simulink model "CryoDetXray"  (R2016b)
settings: Solver=ode45  StartTime=0.0  StopTime=10e-5  MaxStep=Tclk/4  RelTol=1e-3
values from neighbouring files (symbols this model uses):
  Fclk = Fadc    (= 307200000)    [setupCryoFPGAxray.m]
  Tclk = 1/Fclk    (= 3.25520833333e-09)    [setupCryoFPGAxray.m]
undefined symbols (not defined in the file or in its folder): AXI4, Lite, lpf, Naxi, xlipgetpartsetting
libraries: xbsIndex_r4 x1091, CryoDetLib x68, simulink x4, hdlsllib x1
(part 6 of 8)

== system CryoDetXray/DspCore/AdcDac 0/dF1 ==
  note: negate Q component to form conjugate
  note: "Now bandwidth is included in eta'
  note: definition of eta' changed so that now delta(F) = real part of eta'*Sig*conj(Ref)
      | SS 27 Spe 2017
  note: diagnostics
  note: latency 1
  note: pick a channel for diagnostics
  note: sig0
  note: conj(Ref0)
  note: Match latencies
  note: dF1
  note: Ref
  note: Sig
  note: Frequency error dF = Re(eta'*Ref'*Sig)
      | where eta' is like a phase and amplitude calibration including the phase determined by the 2 sidebands and amplitude determined by the reference central line and bandwidth
      |
      | get channel ID
      | fetch eta'
      | calc dF
  note: latency 12
  note: latency 12
  In1 : Inport
  Bus Creator : BusCreator  Inputs=2
  Bus Selector : BusSelector  OutputSignals=channel,Sig&Ref
  Bus Selector1 : BusSelector  OutputSignals=SignalQ&I,ReferenceQ&I
  Bus Selector2 : BusSelector  OutputSignals=refQ,refI
  Bus Selector3 : BusSelector  OutputSignals=sigQ,sigI
  Bus Selector4 : BusSelector  OutputSignals=imEta,reEta
  CMult : xbsIndex_r4/CMult  const=-1  gui_display_data_type=Fixed-point  const_n_bits=16  const_bin_pt=15  float_type=Single  exp_bits=8  fraction_bits=24  en=off  latency=1  precision=User Defined  arith_type="Signed  (2's comp)"  n_bits=16  bin_pt=16  quantization=Truncate  overflow=Saturate  use_behavioral_HDL=on  mem_type=Distributed RAM  pipeline=off  dbl_ovrd=off  block_type=cmult
  Chan Synch scope : Scope  Commented=on  NumInputPorts=2
  "Complex Multiplier 6.0 " : xbsIndex_r4/Complex Multiplier 6.0   hasatlast=off  hasatuser=off  atuserwidth=1  hasbtlast=off  hasbtuser=on  btuserwidth=4  multtype=Use_Mults  optimizegoal=Performance  flowcontrol=NonBlocking  outputwidth=20  roundmode=Truncate  hasctrltlast=off  hasctrltuser=off  ctrltuserwidth=1  outtlastbehv=Null  latencyconfig=Manual  minimumlatency=8  aclken=off  aresetn=off  trim_axipin_name=on  simulation_type=hybrid_sim  simulation_model=sysgen:cmpy_v6_0  data_path_portlist={ 's_axis_a_tdata_real', 's_axis_a_tdata_imag', 's_axis_b_tdata_real', 's_axis_b_tdata_imag', 's_axis_ctrl_tdata_rounding_bit', 'm_axis_dout_tdata_real', 'm_axis_dout_tdata_imag' }  aportwidth=63  bportwidth=63  ip_name=Complex Multiplier  ip_version=6.0  dsptool_ready=true  ipcore_usecache=true  ipcore_useipmodelcache=true  ipcore_verbose=false  ipcore_latency_parameter='minimumlatency'  wrapper_available=true  port_translation_map={ 'aclken' => 'en', 'aresetn' => 'rst'}  block_type=cmpy_v6_0
  Complex Multiplier 6.0 1 : xbsIndex_r4/Complex Multiplier 6.0   hasatlast=off  hasatuser=on  atuserwidth=4  hasbtlast=off  hasbtuser=off  btuserwidth=1  multtype=Use_Mults  optimizegoal=Performance  flowcontrol=NonBlocking  outputwidth=34  roundmode=Truncate  hasctrltlast=off  hasctrltuser=off  ctrltuserwidth=1  outtlastbehv=Null  latencyconfig=Manual  minimumlatency=12  aclken=off  aresetn=off  trim_axipin_name=on  simulation_type=hybrid_sim  simulation_model=sysgen:cmpy_v6_0  data_path_portlist={ 's_axis_a_tdata_real', 's_axis_a_tdata_imag', 's_axis_b_tdata_real', 's_axis_b_tdata_imag', 's_axis_ctrl_tdata_rounding_bit', 'm_axis_dout_tdata_real', 'm_axis_dout_tdata_imag' }  aportwidth=63  bportwidth=63  ip_name=Complex Multiplier  ip_version=6.0  dsptool_ready=true  ipcore_usecache=true  ipcore_useipmodelcache=true  ipcore_verbose=false  ipcore_latency_parameter='minimumlatency'  wrapper_available=true  port_translation_map={ 'aclken' => 'en', 'aresetn' => 'rst'}  block_type=cmpy_v6_0
  Constant : xbsIndex_r4/Constant  const=0  gui_display_data_type=Fixed-point  arith_type=Unsigned  n_bits=4  bin_pt=0  preci_type=Single  exp_width=8  frac_width=24  explicit_period=off  period=1  equ=P=C  opselect=C  inp2=PCIN>>17  opr=+  inp1=P  carry=CIN  dbl_ovrd=off  block_type=constant
  Constant1 : xbsIndex_r4/Constant  const=1  gui_display_data_type=Fixed-point  arith_type=Unsigned  n_bits=4  bin_pt=0  preci_type=Single  exp_width=8  frac_width=24  explicit_period=off  period=1  equ=P=C  opselect=C  inp2=PCIN>>17  opr=+  inp1=P  carry=CIN  dbl_ovrd=off  block_type=constant
  Constant2 : xbsIndex_r4/Constant  const=1.0  gui_display_data_type=Boolean  arith_type=Boolean  n_bits=16  bin_pt=14  preci_type=Single  exp_width=8  frac_width=24  explicit_period=on  period=Tclk  equ=P=C  opselect=C  inp2=PCIN>>17  opr=+  inp1=P  carry=CIN  dbl_ovrd=off  block_type=constant
  Constant3 : xbsIndex_r4/Constant  const=0  gui_display_data_type=Fixed-point  arith_type=Unsigned  n_bits=4  bin_pt=0  preci_type=Single  exp_width=8  frac_width=24  explicit_period=off  period=1  equ=P=C  opselect=C  inp2=PCIN>>17  opr=+  inp1=P  carry=CIN  dbl_ovrd=off  block_type=constant
  Constant4 : Constant  Value=0
  Convert : xbsIndex_r4/Convert  gui_display_data_type=Fixed-point  arith_type="Signed  (2's comp)"  n_bits=16  bin_pt=16  float_type=Single  exp_bits=8  fraction_bits=24  quantization=Truncate  overflow=Wrap  en=off  latency=1  pipeline=on  dbl_ovrd=off  block_type=convert
  Convert1 : xbsIndex_r4/Convert  gui_display_data_type=Fixed-point  arith_type="Signed  (2's comp)"  n_bits=16  bin_pt=16  float_type=Single  exp_bits=8  fraction_bits=24  quantization=Truncate  overflow=Wrap  en=off  latency=1  pipeline=on  dbl_ovrd=off  block_type=convert
  Convert3 : xbsIndex_r4/Convert  gui_display_data_type=Fixed-point  arith_type="Signed  (2's comp)"  n_bits=16  bin_pt=16  float_type=Single  exp_bits=8  fraction_bits=24  quantization=Truncate  overflow=Wrap  en=off  latency=1  pipeline=on  dbl_ovrd=off  block_type=convert
  Convert4 : xbsIndex_r4/Convert  gui_display_data_type=Fixed-point  arith_type="Signed  (2's comp)"  n_bits=32  bin_pt=30  float_type=Single  exp_bits=8  fraction_bits=24  quantization="Round  (unbiased: +/- Inf)"  overflow=Saturate  en=off  latency=1  pipeline=off  dbl_ovrd=off  block_type=convert
  Convert6 : xbsIndex_r4/Convert  gui_display_data_type=Fixed-point  arith_type="Signed  (2's comp)"  n_bits=16  bin_pt=14  float_type=Single  exp_bits=8  fraction_bits=24  quantization=Truncate  overflow=Wrap  en=off  latency=1  pipeline=on  dbl_ovrd=off  block_type=convert
  Convert7 : xbsIndex_r4/Convert  gui_display_data_type=Fixed-point  arith_type="Signed  (2's comp)"  n_bits=16  bin_pt=14  float_type=Single  exp_bits=8  fraction_bits=24  quantization=Truncate  overflow=Wrap  en=off  latency=1  pipeline=on  dbl_ovrd=off  block_type=convert
  Delay{1,5..6,10..11} (5 alike) : xbsIndex_r4/Delay  rst=off  infoeditControl=Selection of Reset will increase slice count due to use of real FFs and instead of SRLs  en=off  latency=1  reg_retiming=on  dbl_ovrd=off  block_type=delay
  Delay3 : xbsIndex_r4/Delay  rst=off  infoeditControl=Selection of Reset will increase slice count due to use of real FFs and instead of SRLs  en=off  latency=12  reg_retiming=on  dbl_ovrd=off  block_type=delay
  Delay4 : xbsIndex_r4/Delay  rst=off  infoeditControl=Selection of Reset will increase slice count due to use of real FFs and instead of SRLs  en=off  latency=6  reg_retiming=on  dbl_ovrd=off  block_type=delay
  Freq Error : Scope
  Gain3 : Gain  Gain=Fclk/1e6
  Gain4 : Gain  Gain=Fclk/1e6
  Gateway Out{1..7,9} (8 alike) : xbsIndex_r4/Gateway Out  inherit_from_input=off  hdl_port=off  rows=1  columns=1  UseAsDAC=off  DACChannel='1'  interface=None  automatic_assignment=on  address_offset=hex2dec('00')  intf_name=''  intf_description=''  timing_constraint=None  locs_specified=off  LOCs={}  io_standard={}  block_type=gatewayout
  Im SigXRef 0 : Display
  Re SigXRef 0 : Display
  Register{,1..3} (4 alike) : xbsIndex_r4/Register  init=0  rst=off  en=on  dbl_ovrd=off  block_type=register
  Register{4..7} (4 alike) : xbsIndex_r4/Register  init=0  rst=off  en=off  dbl_ovrd=off  block_type=register
  Relational : xbsIndex_r4/Relational  mode=a=b  op_type=Bool  en=off  latency=0  dbl_ovrd=off  block_type=relational
  Relational1 : xbsIndex_r4/Relational  mode=a=b  op_type=Bool  en=off  latency=0  dbl_ovrd=off  block_type=relational
  Relational2 : xbsIndex_r4/Relational  mode=a=b  op_type=Bool  en=off  latency=0  dbl_ovrd=off  block_type=relational
  Repeating Sequence : simulink/Sources/Repeating Sequence  rep_seq_t=[0 0.99e-6 1.01e-6 1]  rep_seq_y=[1 1 0 0]
  SigXrefIQ : Scope  NumInputPorts=2
  Switch : Switch  Criteria=u2 > Threshold  Threshold=.5  ZeroCross=off
  Terminator1 : Terminator
  Terminator2 : Terminator
  Terminator3 : Terminator
  "chan 0 " : Display
  chan 1 : Display
  "dF1scope " : Scope  NumInputPorts=3
  eta Mux : Subsystem
  Out1 : Outport
  tag scope: dFbusHBW=global
  wires:
  Bus Selector1/1 -> Bus Selector3/1  "<SignalQ&I>"
  Bus Selector1/2 -> Bus Selector2/1  "<ReferenceQ&I>"
  Bus Selector2/1 -> Register6/1  "<refQ>"
  Bus Selector2/2 -> Register7/1  "<refI>"
  Bus Selector3/2 -> Register5/1  "<sigI>"
  Bus Selector3/1 -> Register4/1  "<sigQ>"
  In1/1 -> Bus Selector/1
  Bus Selector/1 -> Delay10/1  "<channel>"
  Bus Selector/2 -> Bus Selector1/1  "<Sig&Ref>"
  Delay4/1 -> Delay1/1, eta Mux/1(channel)
  Complex Multiplier 6.0 1/3 -> Gateway Out1/1, Convert4/1  "freqError"
  "Complex Multiplier 6.0 "/2 -> Register3/1, Complex Multiplier 6.0 1/2
  "Complex Multiplier 6.0 "/3 -> Register2/1, Complex Multiplier 6.0 1/3
  Bus Selector4/1 -> Convert6/1  "<imEta>"
  Bus Selector4/2 -> Convert7/1  "<reEta>"
  Convert4/1 -> Bus Creator/2, Register1/1, Register/1  "freqError"
  Gateway Out4/1 -> Gain3/1
  Constant/1 -> Relational/2
  Relational/1 -> Register/2
  Register/1 -> Gateway Out4/1
  [BW] -> Terminator3/1
  Bus Creator/1 -> [dFbusHBW], Out1/1
  Delay6/1 -> Bus Creator/1, Relational/1, Relational1/1  "channel"
  Gateway Out2/1 -> Gain4/1
  Constant1/1 -> Relational1/2
  Relational1/1 -> Register1/2
  Register1/1 -> Gateway Out2/1
  eta Mux/1(eta out) -> Bus Selector4/1
  Delay3/1 -> Gateway Out9/1, Delay6/1
  [dFbusHBW] -> Terminator1/1
  Convert6/1 -> Complex Multiplier 6.0 1/6
  Convert7/1 -> Complex Multiplier 6.0 1/7
  Gain4/1 -> chan 1/1
  Gain3/1 -> Switch/3, "chan 0 "/1
  Delay5/1 -> Delay3/1, Relational2/1
  Constant3/1 -> Relational2/2
  Relational2/1 -> Register2/2, Register3/2
  Register2/1 -> Gateway Out5/1
  Gateway Out5/1 -> SigXrefIQ/1, Re SigXRef 0/1
  Gateway Out6/1 -> SigXrefIQ/2, Im SigXRef 0/1
  Register3/1 -> Gateway Out6/1
  Switch/1 -> Freq Error/1
  Repeating Sequence/1 -> Switch/2
  Constant4/1 -> Switch/1
  Complex Multiplier 6.0 1/2 -> Gateway Out3/1
  Register4/1 -> Convert/1
  Delay10/1 -> Delay11/1
  Register5/1 -> Convert1/1
  Delay11/1 -> "Complex Multiplier 6.0 "/7, Delay4/1
  Delay1/1 -> Delay5/1
  Convert/1 -> "Complex Multiplier 6.0 "/2
  Convert1/1 -> "Complex Multiplier 6.0 "/3
  Constant2/1 -> "Complex Multiplier 6.0 "/4, "Complex Multiplier 6.0 "/1
  "Complex Multiplier 6.0 "/1 -> Complex Multiplier 6.0 1/5, Complex Multiplier 6.0 1/1
  "Complex Multiplier 6.0 "/4 -> Complex Multiplier 6.0 1/4
  Complex Multiplier 6.0 1/1 -> Terminator2/1
  CMult/1 -> "Complex Multiplier 6.0 "/5
  Convert3/1 -> "Complex Multiplier 6.0 "/6
  Complex Multiplier 6.0 1/4 -> Gateway Out7/1
  Gateway Out9/1 -> Chan Synch scope/2
  Gateway Out7/1 -> "dF1scope "/3, Chan Synch scope/1
  Gateway Out1/1 -> "dF1scope "/2
  Gateway Out3/1 -> "dF1scope "/1
  Register7/1 -> Convert3/1
  Register6/1 -> CMult/1

== system CryoDetXray/DspCore/AdcDac 0/dphi ==
  note: scale by 1/2 since phase increment per 1/614 = 1/2 of phase increment per 1/307.2 MSPS
  note: dPhi
      | calculate complex phase advance for a single sample of ADC input
      | at the frequency of a single channel and send off on dphiBus
  In1 : Inport
  Bus Creator : BusCreator  Inputs=3
  Bus Selector : BusSelector  OutputSignals=channel,freq
  Constant : xbsIndex_r4/Constant  const=1  gui_display_data_type=Boolean  arith_type=Boolean  n_bits=16  bin_pt=14  preci_type=Single  exp_width=8  frac_width=24  explicit_period=off  period=1  equ=P=C  opselect=C  inp2=PCIN>>17  opr=+  inp1=P  carry=CIN  dbl_ovrd=off  block_type=constant
  Convert : xbsIndex_r4/Convert  gui_display_data_type=Fixed-point  arith_type=Unsigned  n_bits=16  bin_pt=15  float_type=Single  exp_bits=8  fraction_bits=24  quantization="Round  (unbiased: Even Values)"  overflow=Wrap  en=off  latency=1  pipeline=off  dbl_ovrd=off  block_type=convert
  "DDS Compiler 6.0 " : xbsIndex_r4/DDS Compiler 6.0   partspresent=SIN_COS_LUT_only  dds_clock_rate=100  channels=1  mode_of_operation=Standard  modulus=9  parameter_entry=Hardware_Parameters  spurious_free_dynamic_range=45  frequency_resolution=0.4  noise_shaping=None  phase_width=16  output_width=IQbits  output_selection=Sine_and_Cosine  negative_sine=off  negative_cosine=off  amplitude_mode=Unit_Circle  memory_type=Auto  optimization_goal=Speed  dsp48_use=Maximal  resync=off  latency_configuration=Auto  latency=15  has_phase_out=off  has_aclken=off  has_aresetn=off  explicit_period=on  period=Tclk  data_has_tlast=Not_Required  has_tready=off  s_phase_has_tuser=Not_Required  m_data_has_tuser=Not_Required  m_phase_has_tuser=Not_Required  s_phase_tuser_width=1  output_form=Twos_Complement  s_config_sync_mode=On_Vector  phase_increment=Fixed  output_frequency1=0  output_frequency2=0  output_frequency3=0  output_frequency4=0  output_frequency5=0  output_frequency6=0  output_frequency7=0  output_frequency8=0  output_frequency9=0  output_frequency10=0  output_frequency11=0  output_frequency12=0  output_frequency13=0  output_frequency14=0  output_frequency15=0  output_frequency16=0  pinc1='0'  pinc2='0'  pinc3='0'  pinc4='0'  pinc5='0'  pinc6='0'  pinc7='0'  pinc8='0'  pinc9='0'  pinc10='0'  pinc11='0'  pinc12='0'  pinc13='0'  pinc14='0'  pinc15='0'  pinc16='0'  phase_offset=Programmable  phase_offset_angles1=0  phase_offset_angles2=0  phase_offset_angles3=0  phase_offset_angles4=0  phase_offset_angles5=0  phase_offset_angles6=0  phase_offset_angles7=0  phase_offset_angles8=0  phase_offset_angles9=0  phase_offset_angles10=0  phase_offset_angles11=0  phase_offset_angles12=0  phase_offset_angles13=0  phase_offset_angles14=0  phase_offset_angles15=0  phase_offset_angles16=0  poff1='0'  poff2='0'  poff3='0'  poff4='0'  poff5='0'  poff6='0'  poff7='0'  poff8='0'  poff9='0'  poff10='0'  poff11='0'  poff12='0'  poff13='0'  poff14='0'  poff15='0'  poff16='0'  trim_axipin_name=on  simulation_type=hybrid_sim  simulation_model=sysgen:xddsv6_0_cmodel  data_path_portlist={ 's_axis_config_tdata_poff', 's_axis_config_tdata_chan0_poff', 's_axis_config_tdata_pinc', 's_axis_config_tdata_chan0_pinc', 's_axis_phase_tdata_resync', 's_axis_phase_tdata_chan0_resync', 's_axis_phase_tdata_poff', 's_axis_phase_tdata_chan0_poff', 's_axis_phase_tdata_pinc', 's_axis_phase_tdata_chan0_pinc', 's_axis_phase_tdata_phase_in', 'm_axis_data_tdata_sine', 'm_axis_data_tdata_chan0_sine', 'm_axis_data_tdata_cosine', 'm_axis_data_tdata_chan0_cosine', 'm_axis_phase_tdata_phase_out', 'm_axis_phase_tdata_chan0_phase_out'}  por_mode=false  gui_behaviour=Sysgen  ip_name=DDS Compiler  ip_version=6.0  dsptool_ready=true  wrapper_available=true  port_translation_map={ 'aclken' => 'en', 'aresetn' => 'rst' }  ipcore_usecache=true  ipcore_useipmodelcache=true  ipcore_xco_need_fpga_part=true  ipcore_fpga_part=xlipgetpartsetting(gcb, {'kintex7', 'xc7k325t', '-3', 'fbg676'})  ipcore_verbose=false  block_type=dds_compiler_v6_0
  Delay : xbsIndex_r4/Delay  rst=off  infoeditControl=Selection of Reset will increase slice count due to use of real FFs and instead of SRLs  en=off  latency=7  reg_retiming=off  dbl_ovrd=off  block_type=delay
  Display : Display  Commented=on
  Display1 : Display  Commented=on
  Display2 : Display  Commented=on
  Gateway Out : xbsIndex_r4/Gateway Out  Commented=on  inherit_from_input=off  hdl_port=off  rows=1  columns=1  UseAsDAC=off  DACChannel='1'  interface=None  automatic_assignment=on  address_offset=hex2dec('00')  intf_name=''  intf_description=''  timing_constraint=None  locs_specified=off  LOCs={}  io_standard={}  block_type=gatewayout
  Gateway Out1 : xbsIndex_r4/Gateway Out  Commented=on  inherit_from_input=off  hdl_port=off  rows=1  columns=1  UseAsDAC=off  DACChannel='1'  interface=None  automatic_assignment=on  address_offset=hex2dec('00')  intf_name=''  intf_description=''  timing_constraint=None  locs_specified=off  LOCs={}  io_standard={}  block_type=gatewayout
  Gateway Out2 : xbsIndex_r4/Gateway Out  Commented=on  inherit_from_input=off  hdl_port=off  rows=1  columns=1  UseAsDAC=off  DACChannel='1'  interface=None  automatic_assignment=on  address_offset=hex2dec('00')  intf_name=''  intf_description=''  timing_constraint=None  locs_specified=off  LOCs={}  io_standard={}  block_type=gatewayout
  Register1 : xbsIndex_r4/Register  init=0  rst=off  en=off  dbl_ovrd=off  block_type=register
  Register2 : xbsIndex_r4/Register  init=0  rst=off  en=off  dbl_ovrd=off  block_type=register
  Register3 : xbsIndex_r4/Register  init=0  rst=off  en=off  dbl_ovrd=off  block_type=register
  Scale : xbsIndex_r4/Scale  scale_factor=-1  dbl_ovrd=off  block_type=scale
  Terminator : Terminator
  tag scope: dphiBus=global
  wires:
  Bus Creator/1 -> [dphiBus]
  Bus Selector/2 -> Convert/1  "<freq>"
  Delay/1 -> Register1/1  "channel"
  Convert/1 -> Scale/1
  Constant/1 -> "DDS Compiler 6.0 "/1
  "DDS Compiler 6.0 "/2 -> Register2/1, Gateway Out/1  "dPhiQ"
  "DDS Compiler 6.0 "/3 -> Register3/1, Gateway Out1/1  "dPhiI"
  Gateway Out/1 -> Display/1
  Gateway Out1/1 -> Display1/1
  Gateway Out2/1 -> Display2/1
  Bus Selector/1 -> Delay/1  "<channel>"
  "DDS Compiler 6.0 "/1 -> Terminator/1
  In1/1 -> Bus Selector/1
  Scale/1 -> "DDS Compiler 6.0 "/2
  Register1/1 -> Bus Creator/1, Gateway Out2/1  "channel"
  Register2/1 -> Bus Creator/2  "dPhiQ"
  Register3/1 -> Bus Creator/3  "dPhiI"

== system CryoDetXray/DspCore/AdcDac 0/loopFilter1 ==
  note: Just sweep fluxramp phase
  note: reset loop
  note: Hold phase shift
      | if FF not eneabled
  note: diagnostic
  note: Assumes 12 channels processed on sucessive clocks
  note: get enable bit for this channel
  note: diagnostics
  note: flux Ramp Phase Feedback loop Filter
      | multi-line fluxramp Phase feedback block
      | integrator, gain, enable
  In1 : Inport
  AddSub : xbsIndex_r4/AddSub  mode=Addition  use_carryin=off  use_carryout=off  en=off  latency=3  precision=User Defined  arith_type="Signed  (2's comp)"  n_bits=20  bin_pt=18  quantization=Truncate  overflow=Wrap  use_behavioral_HDL=off  hw_selection=Fabric  pipelined=off  dbl_ovrd=off  block_type=addsub
  Bus Creator : BusCreator  Inputs=2
  Bus Selector : BusSelector  OutputSignals=channel,fluxRampQ
  Constant : xbsIndex_r4/Constant  const=0  gui_display_data_type=Fixed-point  arith_type=Unsigned  n_bits=4  bin_pt=0  preci_type=Single  exp_width=8  frac_width=24  explicit_period=off  period=1  equ=P=C  opselect=C  inp2=PCIN>>17  opr=+  inp1=P  carry=CIN  dbl_ovrd=off  block_type=constant
  Constant1 : xbsIndex_r4/Constant  const=0  gui_display_data_type=Fixed-point  arith_type=Unsigned  n_bits=4  bin_pt=0  preci_type=Single  exp_width=8  frac_width=24  explicit_period=off  period=1  equ=P=C  opselect=C  inp2=PCIN>>17  opr=+  inp1=P  carry=CIN  dbl_ovrd=off  block_type=constant
  Constant2 : xbsIndex_r4/Constant  const=1  gui_display_data_type=Fixed-point  arith_type=Unsigned  n_bits=4  bin_pt=0  preci_type=Single  exp_width=8  frac_width=24  explicit_period=off  period=1  equ=P=C  opselect=C  inp2=PCIN>>17  opr=+  inp1=P  carry=CIN  dbl_ovrd=off  block_type=constant
  Constant3 : xbsIndex_r4/Constant  const=0  gui_display_data_type=Fixed-point  arith_type=Unsigned  n_bits=16  bin_pt=16  preci_type=Single  exp_width=8  frac_width=24  explicit_period=off  period=1  equ=P=C  opselect=C  inp2=PCIN>>17  opr=+  inp1=P  carry=CIN  dbl_ovrd=off  block_type=constant
  Convert : xbsIndex_r4/Convert  gui_display_data_type=Fixed-point  arith_type="Signed  (2's comp)"  n_bits=16  bin_pt=16  float_type=Single  exp_bits=8  fraction_bits=24  quantization=Truncate  overflow=Wrap  en=off  latency=0  pipeline=off  dbl_ovrd=off  block_type=convert
  Counter : xbsIndex_r4/Counter  cnt_type=Free Running  cnt_to=Inf  operation=Up  start_count=12000  cnt_by_val=4  arith_type=Unsigned  n_bits=16  bin_pt=0  load_pin=off  rst=off  en=off  explicit_period=on  period=Tclk  use_behavioral_HDL=off  implementation=Fabric  dbl_ovrd=off  block_type=counter
  Delay1 : xbsIndex_r4/Delay  rst=off  infoeditControl=Selection of Reset will increase slice count due to use of real FFs and instead of SRLs  en=off  latency=11  reg_retiming=off  dbl_ovrd=off  block_type=delay
  Delay{2..4,6} (4 alike) : xbsIndex_r4/Delay  rst=off  infoeditControl=Selection of Reset will increase slice count due to use of real FFs and instead of SRLs  en=off  latency=3  reg_retiming=off  dbl_ovrd=off  block_type=delay
  Delay5 : xbsIndex_r4/Delay  rst=off  infoeditControl=Selection of Reset will increase slice count due to use of real FFs and instead of SRLs  en=off  latency=1  reg_retiming=off  dbl_ovrd=off  block_type=delay
  Delay7 : xbsIndex_r4/Delay  rst=off  infoeditControl=Selection of Reset will increase slice count due to use of real FFs and instead of SRLs  en=off  latency=1  reg_retiming=off  dbl_ovrd=off  block_type=delay
  Display{1..6} (6 alike) : Display
  Gateway Out1 : xbsIndex_r4/Gateway Out  inherit_from_input=on  hdl_port=off  rows=1  columns=1  UseAsDAC=off  DACChannel='1'  interface=None  automatic_assignment=on  address_offset=hex2dec('00')  intf_name=''  intf_description=''  timing_constraint=None  locs_specified=off  LOCs={}  io_standard={}  block_type=gatewayout
  Gateway Out{2..4,6..10,12} (9 alike) : xbsIndex_r4/Gateway Out  inherit_from_input=off  hdl_port=off  rows=1  columns=1  UseAsDAC=off  DACChannel='1'  interface=None  automatic_assignment=on  address_offset=hex2dec('00')  intf_name=''  intf_description=''  timing_constraint=None  locs_specified=off  LOCs={}  io_standard={}  block_type=gatewayout
  Gateway Out13 : xbsIndex_r4/Gateway Out  inherit_from_input=on  hdl_port=off  rows=1  columns=1  UseAsDAC=off  DACChannel='1'  interface=None  automatic_assignment=on  address_offset=hex2dec('00')  intf_name=''  intf_description=''  timing_constraint=None  locs_specified=off  LOCs={}  io_standard={}  block_type=gatewayout
  Gateway Out5 : xbsIndex_r4/Gateway Out  inherit_from_input=on  hdl_port=off  rows=1  columns=1  UseAsDAC=off  DACChannel='1'  interface=None  automatic_assignment=on  address_offset=hex2dec('00')  intf_name=''  intf_description=''  timing_constraint=None  locs_specified=off  LOCs={}  io_standard={}  block_type=gatewayout
  Logical : xbsIndex_r4/Logical  logical_function=AND  inputs=2  en=off  latency=0  precision=User Defined  arith_type=Unsigned  n_bits=1  bin_pt=0  align_bp=on  dbl_ovrd=off  block_type=logical
  Loop filter scope : Scope  NumInputPorts=3
  Mult : xbsIndex_r4/Mult  precision=User Defined  arith_type="Signed  (2's comp)"  n_bits=32  bin_pt=30  quantization=Truncate  overflow=Saturate  en=off  latency=3  use_behavioral_HDL=off  opt=Speed  use_embedded=on  optimum_pipeline=off  pipeline=on  dbl_ovrd=off  use_rpm=on  placement_style=Triangular  block_type=mult
  Mux : xbsIndex_r4/Mux  inputs=2  en=off  latency=1  precision=User Defined  arith_type="Signed  (2's comp)"  n_bits=17  bin_pt=4  quantization=Truncate  overflow=Wrap  dbl_ovrd=off  block_type=mux
  Mux1 : xbsIndex_r4/Mux  inputs=2  en=off  latency=1  precision=User Defined  arith_type="Signed  (2's comp)"  n_bits=20  bin_pt=18  quantization=Truncate  overflow=Wrap  dbl_ovrd=off  block_type=mux
  Mux3 : xbsIndex_r4/Mux  inputs=2  en=off  latency=1  precision=User Defined  arith_type="Signed  (2's comp)"  n_bits=20  bin_pt=18  quantization=Truncate  overflow=Wrap  dbl_ovrd=off  block_type=mux
  Negate : xbsIndex_r4/Negate  precision=Full  arith_type=Unsigned  n_bits=17  bin_pt=12  quantization=Truncate  overflow=Wrap  en=off  latency=1  dbl_ovrd=off  block_type=negate
  Register : xbsIndex_r4/Register  init=0  rst=off  en=on  dbl_ovrd=off  block_type=register
  Register1 : xbsIndex_r4/Register  init=0  rst=off  en=on  dbl_ovrd=off  block_type=register
  Register2 : xbsIndex_r4/Register  init=0  rst=off  en=on  dbl_ovrd=off  block_type=register
  Relational : xbsIndex_r4/Relational  mode=a=b  op_type=Bool  en=off  latency=0  dbl_ovrd=off  block_type=relational
  Relational1 : xbsIndex_r4/Relational  mode=a=b  op_type=Bool  en=off  latency=0  dbl_ovrd=off  block_type=relational
  Relational2 : xbsIndex_r4/Relational  mode=a=b  op_type=Bool  en=off  latency=0  dbl_ovrd=off  block_type=relational
  Scale : xbsIndex_r4/Scale  scale_factor=-16  dbl_ovrd=off  block_type=scale
  Slice : xbsIndex_r4/Slice  nbits=1  boolean_output=on  mode=Lower Bit Location + Width  bit1=0  base1=MSB of Input  bit0=24  base0=LSB of Input  dbl_ovrd=off  block_type=slice
  Terminator : Terminator
  "chan 0 " : Display
  chan 1 : Display
  initial Frequencies : Subsystem
  loop filter input : Scope  NumInputPorts=4
  loop filter output : Scope  NumInputPorts=4
  Out1 : Outport
  wires:
  In1/1 -> Bus Selector/1
  Bus Selector/1 -> Relational/1, Gateway Out3/1, Delay3/1  "<channel>"
  Bus Selector/2 -> Mult/1, Gateway Out9/1, Register/1  "<fluxRampQ>"
  Delay3/1 -> Delay2/1, initial Frequencies/1(channel)  "channel"
  Mux1/1 -> Gateway Out2/1, Gateway Out7/1, Delay1/1, Convert/1
  Bus Creator/1 -> Out1/1
  [FFpolarity] -> Mux/1
  [FFgain] -> Negate/1, Mux/2, Gateway Out10/1
  initial Frequencies/1(Fi) -> Slice/1
  Gateway Out12/1 -> loop filter output/1
  Gateway Out3/1 -> loop filter input/1, Display2/1
  Constant/1 -> Relational/2
  Relational/1 -> Register/2
  Register/1 -> Gateway Out4/1
  Constant1/1 -> Relational1/1
  Relational1/1 -> Register1/2
  Register1/1 -> Gateway Out13/1
  Gateway Out13/1 -> Display4/1, loop filter output/2
  Gateway Out4/1 -> Display3/1, loop filter input/2
  Constant2/1 -> Relational2/1
  Relational2/1 -> Register2/2
  Register2/1 -> Gateway Out5/1
  Gateway Out5/1 -> Display1/1, loop filter output/3
  Negate/1 -> Mux/3
  Mux/1 -> Mult/2
  Gateway Out1/1 -> loop filter output/4
  Mult/1 -> Gateway Out6/1, AddSub/1
  Delay1/1 -> AddSub/2, Delay6/1
  Slice/1 -> Delay4/1
  [FBen] -> Logical/1
  Gateway Out7/1 -> "chan 0 "/1, Loop filter scope/2
  Gateway Out6/1 -> Display5/1, Loop filter scope/1
  Gateway Out2/1 -> chan 1/1, Loop filter scope/3
  Gateway Out9/1 -> loop filter input/3
  Gateway Out10/1 -> loop filter input/4
  Delay2/1 -> Delay7/1
  Delay4/1 -> Logical/2
  Delay5/1 -> Bus Creator/1, Relational2/2, Gateway Out12/1, Relational1/2  "channel"
  Logical/1 -> Mux3/1
  [fpgaReset] -> Mux1/1
  AddSub/1 -> Mux3/3
  Delay6/1 -> Mux3/2
  Constant3/1 -> Mux1/3
  Delay7/1 -> Delay5/1
  Convert/1 -> Gateway Out8/1, Bus Creator/2, Gateway Out1/1, Register2/1, Register1/1  "fluxRampPhaseShift"
  Mux3/1 -> Mux1/2
  Counter/1 -> Scale/1  "fluxRampPhaseShift"
  Gateway Out8/1 -> Display6/1
  Scale/1 -> Terminator/1  "fluxRampPhaseShift"

== system CryoDetXray/DspCore/AdcDac 0/shiftFreq ==
  note: Frequency shift interleaved complex DAC drive signals
  note: for now use another entire DDS to generate odd samples of LO
      | eventaully copy dPhi scheme of using one DDS to generate complex phase increment for all 16 sub-bands
      | creating another equivalent of dPhiBus
      |
      | Eventaully will sum 2 sub-bands to one DAC channel
      | at which time there will be 2 frequency translation stages followed by sums for Q0, I0, Q1, I1
  In1 : Inport
  Bus Creator : BusCreator  Inputs=4
  Bus Selector : BusSelector  OutputSignals=Q0,I0,Q1,I1
  "Complex Multiplier 6.0 " : xbsIndex_r4/Complex Multiplier 6.0   hasatlast=off  hasatuser=off  atuserwidth=1  hasbtlast=off  hasbtuser=off  btuserwidth=1  multtype=Use_Mults  optimizegoal=Resources  flowcontrol=NonBlocking  outputwidth=19  roundmode=Truncate  hasctrltlast=off  hasctrltuser=off  ctrltuserwidth=1  outtlastbehv=Null  latencyconfig=Automatic  minimumlatency=37  aclken=off  aresetn=off  trim_axipin_name=on  simulation_type=hybrid_sim  simulation_model=sysgen:cmpy_v6_0  data_path_portlist={ 's_axis_a_tdata_real', 's_axis_a_tdata_imag', 's_axis_b_tdata_real', 's_axis_b_tdata_imag', 's_axis_ctrl_tdata_rounding_bit', 'm_axis_dout_tdata_real', 'm_axis_dout_tdata_imag' }  aportwidth=63  bportwidth=63  ip_name=Complex Multiplier  ip_version=6.0  dsptool_ready=true  ipcore_usecache=true  ipcore_useipmodelcache=true  ipcore_verbose=false  ipcore_latency_parameter='minimumlatency'  wrapper_available=true  port_translation_map={ 'aclken' => 'en', 'aresetn' => 'rst'}  block_type=cmpy_v6_0
  Complex Multiplier 6.0 1 : xbsIndex_r4/Complex Multiplier 6.0   hasatlast=off  hasatuser=off  atuserwidth=1  hasbtlast=off  hasbtuser=off  btuserwidth=1  multtype=Use_Mults  optimizegoal=Resources  flowcontrol=NonBlocking  outputwidth=19  roundmode=Truncate  hasctrltlast=off  hasctrltuser=off  ctrltuserwidth=1  outtlastbehv=Null  latencyconfig=Automatic  minimumlatency=37  aclken=off  aresetn=off  trim_axipin_name=on  simulation_type=hybrid_sim  simulation_model=sysgen:cmpy_v6_0  data_path_portlist={ 's_axis_a_tdata_real', 's_axis_a_tdata_imag', 's_axis_b_tdata_real', 's_axis_b_tdata_imag', 's_axis_ctrl_tdata_rounding_bit', 'm_axis_dout_tdata_real', 'm_axis_dout_tdata_imag' }  aportwidth=63  bportwidth=63  ip_name=Complex Multiplier  ip_version=6.0  dsptool_ready=true  ipcore_usecache=true  ipcore_useipmodelcache=true  ipcore_verbose=false  ipcore_latency_parameter='minimumlatency'  wrapper_available=true  port_translation_map={ 'aclken' => 'en', 'aresetn' => 'rst'}  block_type=cmpy_v6_0
  Constant : xbsIndex_r4/Constant  const=1  gui_display_data_type=Boolean  arith_type=Boolean  n_bits=16  bin_pt=14  preci_type=Single  exp_width=8  frac_width=24  explicit_period=off  period=1  equ=P=C  opselect=C  inp2=PCIN>>17  opr=+  inp1=P  carry=CIN  dbl_ovrd=off  block_type=constant
  Constant1 : xbsIndex_r4/Constant  const=1  gui_display_data_type=Boolean  arith_type=Boolean  n_bits=16  bin_pt=14  preci_type=Single  exp_width=8  frac_width=24  explicit_period=off  period=1  equ=P=C  opselect=C  inp2=PCIN>>17  opr=+  inp1=P  carry=CIN  dbl_ovrd=off  block_type=constant
  Convert{,1..3} (4 alike) : xbsIndex_r4/Convert  gui_display_data_type=Fixed-point  arith_type="Signed  (2's comp)"  n_bits=16  bin_pt=15  float_type=Single  exp_bits=8  fraction_bits=24  quantization=Truncate  overflow=Wrap  en=off  latency=1  pipeline=off  dbl_ovrd=off  block_type=convert
  DAC drive : Scope  Commented=on  NumInputPorts=4
  "DDS Compiler 6.0 " : xbsIndex_r4/DDS Compiler 6.0   partspresent=Phase_Generator_and_SIN_COS_LUT  dds_clock_rate=Fclk/1e6  channels=1  mode_of_operation=Standard  modulus=9  parameter_entry=Hardware_Parameters  spurious_free_dynamic_range=45  frequency_resolution=0.4  noise_shaping=None  phase_width=16  output_width=12  output_selection=Sine_and_Cosine  negative_sine=off  negative_cosine=off  amplitude_mode=Unit_Circle  memory_type=Auto  optimization_goal=Speed  dsp48_use=Maximal  resync=off  latency_configuration=Configurable  latency=15  has_phase_out=off  has_aclken=off  has_aresetn=off  explicit_period=on  period=Tclk  data_has_tlast=Not_Required  has_tready=off  s_phase_has_tuser=Not_Required  m_data_has_tuser=Not_Required  m_phase_has_tuser=Not_Required  s_phase_tuser_width=1  output_form=Twos_Complement  s_config_sync_mode=On_Vector  phase_increment=Programmable  output_frequency1=0  output_frequency2=0  output_frequency3=0  output_frequency4=0  output_frequency5=0  output_frequency6=0  output_frequency7=0  output_frequency8=0  output_frequency9=0  output_frequency10=0  output_frequency11=0  output_frequency12=0  output_frequency13=0  output_frequency14=0  output_frequency15=0  output_frequency16=0  pinc1='0'  pinc2='0'  pinc3='0'  pinc4='0'  pinc5='0'  pinc6='0'  pinc7='0'  pinc8='0'  pinc9='0'  pinc10='0'  pinc11='0'  pinc12='0'  pinc13='0'  pinc14='0'  pinc15='0'  pinc16='0'  phase_offset=None  phase_offset_angles1=0  phase_offset_angles2=0  phase_offset_angles3=0  phase_offset_angles4=0  phase_offset_angles5=0  phase_offset_angles6=0  phase_offset_angles7=0  phase_offset_angles8=0  phase_offset_angles9=0  phase_offset_angles10=0  phase_offset_angles11=0  phase_offset_angles12=0  phase_offset_angles13=0  phase_offset_angles14=0  phase_offset_angles15=0  phase_offset_angles16=0  poff1='0'  poff2='0'  poff3='0'  poff4='0'  poff5='0'  poff6='0'  poff7='0'  poff8='0'  poff9='0'  poff10='0'  poff11='0'  poff12='0'  poff13='0'  poff14='0'  poff15='0'  poff16='0'  trim_axipin_name=on  simulation_type=hybrid_sim  simulation_model=sysgen:xddsv6_0_cmodel  data_path_portlist={ 's_axis_config_tdata_poff', 's_axis_config_tdata_chan0_poff', 's_axis_config_tdata_pinc', 's_axis_config_tdata_chan0_pinc', 's_axis_phase_tdata_resync', 's_axis_phase_tdata_chan0_resync', 's_axis_phase_tdata_poff', 's_axis_phase_tdata_chan0_poff', 's_axis_phase_tdata_pinc', 's_axis_phase_tdata_chan0_pinc', 's_axis_phase_tdata_phase_in', 'm_axis_data_tdata_sine', 'm_axis_data_tdata_chan0_sine', 'm_axis_data_tdata_cosine', 'm_axis_data_tdata_chan0_cosine', 'm_axis_phase_tdata_phase_out', 'm_axis_phase_tdata_chan0_phase_out'}  por_mode=false  gui_behaviour=Sysgen  ip_name=DDS Compiler  ip_version=6.0  dsptool_ready=true  wrapper_available=true  port_translation_map={ 'aclken' => 'en', 'aresetn' => 'rst' }  ipcore_usecache=true  ipcore_useipmodelcache=true  ipcore_xco_need_fpga_part=true  ipcore_fpga_part=xlipgetpartsetting(gcb, {'kintex7', 'xc7k325t', '-3', 'fbg676'})  ipcore_verbose=false  block_type=dds_compiler_v6_0
  DDS Compiler 6.0 1 : xbsIndex_r4/DDS Compiler 6.0   partspresent=Phase_Generator_and_SIN_COS_LUT  dds_clock_rate=Fclk/1e6  channels=1  mode_of_operation=Standard  modulus=9  parameter_entry=Hardware_Parameters  spurious_free_dynamic_range=45  frequency_resolution=0.4  noise_shaping=None  phase_width=16  output_width=12  output_selection=Sine_and_Cosine  negative_sine=off  negative_cosine=off  amplitude_mode=Unit_Circle  memory_type=Auto  optimization_goal=Speed  dsp48_use=Maximal  resync=off  latency_configuration=Configurable  latency=15  has_phase_out=off  has_aclken=off  has_aresetn=off  explicit_period=on  period=Tclk  data_has_tlast=Not_Required  has_tready=off  s_phase_has_tuser=Not_Required  m_data_has_tuser=Not_Required  m_phase_has_tuser=Not_Required  s_phase_tuser_width=1  output_form=Twos_Complement  s_config_sync_mode=On_Vector  phase_increment=Programmable  output_frequency1=0  output_frequency2=0  output_frequency3=0  output_frequency4=0  output_frequency5=0  output_frequency6=0  output_frequency7=0  output_frequency8=0  output_frequency9=0  output_frequency10=0  output_frequency11=0  output_frequency12=0  output_frequency13=0  output_frequency14=0  output_frequency15=0  output_frequency16=0  pinc1='0'  pinc2='0'  pinc3='0'  pinc4='0'  pinc5='0'  pinc6='0'  pinc7='0'  pinc8='0'  pinc9='0'  pinc10='0'  pinc11='0'  pinc12='0'  pinc13='0'  pinc14='0'  pinc15='0'  pinc16='0'  phase_offset=Programmable  phase_offset_angles1=0  phase_offset_angles2=0  phase_offset_angles3=0  phase_offset_angles4=0  phase_offset_angles5=0  phase_offset_angles6=0  phase_offset_angles7=0  phase_offset_angles8=0  phase_offset_angles9=0  phase_offset_angles10=0  phase_offset_angles11=0  phase_offset_angles12=0  phase_offset_angles13=0  phase_offset_angles14=0  phase_offset_angles15=0  phase_offset_angles16=0  poff1='0'  poff2='0'  poff3='0'  poff4='0'  poff5='0'  poff6='0'  poff7='0'  poff8='0'  poff9='0'  poff10='0'  poff11='0'  poff12='0'  poff13='0'  poff14='0'  poff15='0'  poff16='0'  trim_axipin_name=on  simulation_type=hybrid_sim  simulation_model=sysgen:xddsv6_0_cmodel  data_path_portlist={ 's_axis_config_tdata_poff', 's_axis_config_tdata_chan0_poff', 's_axis_config_tdata_pinc', 's_axis_config_tdata_chan0_pinc', 's_axis_phase_tdata_resync', 's_axis_phase_tdata_chan0_resync', 's_axis_phase_tdata_poff', 's_axis_phase_tdata_chan0_poff', 's_axis_phase_tdata_pinc', 's_axis_phase_tdata_chan0_pinc', 's_axis_phase_tdata_phase_in', 'm_axis_data_tdata_sine', 'm_axis_data_tdata_chan0_sine', 'm_axis_data_tdata_cosine', 'm_axis_data_tdata_chan0_cosine', 'm_axis_phase_tdata_phase_out', 'm_axis_phase_tdata_chan0_phase_out'}  por_mode=false  gui_behaviour=Sysgen  ip_name=DDS Compiler  ip_version=6.0  dsptool_ready=true  wrapper_available=true  port_translation_map={ 'aclken' => 'en', 'aresetn' => 'rst' }  ipcore_usecache=true  ipcore_useipmodelcache=true  ipcore_xco_need_fpga_part=true  ipcore_fpga_part=xlipgetpartsetting(gcb, {'kintex7', 'xc7k325t', '-3', 'fbg676'})  ipcore_verbose=false  block_type=dds_compiler_v6_0
  Gateway Out{,1..3,6..9} (8 alike) : xbsIndex_r4/Gateway Out  Commented=on  inherit_from_input=off  hdl_port=off  rows=1  columns=1  UseAsDAC=off  DACChannel='1'  interface=None  automatic_assignment=on  address_offset=hex2dec('00')  intf_name=''  intf_description=''  timing_constraint=None  locs_specified=off  LOCs={}  io_standard={}  block_type=gatewayout
  Mux : Mux  Commented=on  Inputs=2
  Mux1 : Mux  Commented=on  Inputs=2
  Scope : Scope  Commented=on  NumInputPorts=2
  Shift : xbsIndex_r4/Shift  shift_dir=Right  shift_bits=1  en=off  latency=1  precision=User Defined  arith_type=Unsigned  n_bits=16  bin_pt=16  quantization=Truncate  overflow=Wrap  dbl_ovrd=off  block_type=shift
  Out1 : Outport
  wires:
  In1/1 -> Bus Selector/1
  [fShift0] -> "DDS Compiler 6.0 "/2, Shift/1, DDS Compiler 6.0 1/3
  Constant/1 -> DDS Compiler 6.0 1/1, "DDS Compiler 6.0 "/1
  "DDS Compiler 6.0 "/2 -> Gateway Out1/1, "Complex Multiplier 6.0 "/5
  "DDS Compiler 6.0 "/3 -> Gateway Out/1, "Complex Multiplier 6.0 "/6
  DDS Compiler 6.0 1/3 -> Gateway Out2/1, Complex Multiplier 6.0 1/6
  DDS Compiler 6.0 1/2 -> Gateway Out3/1, Complex Multiplier 6.0 1/5
  Bus Selector/1 -> Gateway Out6/1, "Complex Multiplier 6.0 "/2  "<Q0>"
  Bus Selector/2 -> Gateway Out7/1, "Complex Multiplier 6.0 "/3  "<I0>"
  Constant1/1 -> "Complex Multiplier 6.0 "/1, Complex Multiplier 6.0 1/1
  Bus Selector/3 -> Gateway Out8/1, Complex Multiplier 6.0 1/2  "<Q1>"
  Bus Selector/4 -> Gateway Out9/1, Complex Multiplier 6.0 1/3  "<I1>"
  "Complex Multiplier 6.0 "/2 -> Convert/1  "Q0"
  "Complex Multiplier 6.0 "/3 -> Convert1/1  "I0"
  Complex Multiplier 6.0 1/2 -> Convert2/1  "Q1"
  Complex Multiplier 6.0 1/3 -> Convert3/1  "I1"
  DDS Compiler 6.0 1/1 -> Complex Multiplier 6.0 1/4
  "DDS Compiler 6.0 "/1 -> "Complex Multiplier 6.0 "/4
  Bus Creator/1 -> Out1/1
  Convert/1 -> Bus Creator/1  "Q0"
  Convert1/1 -> Bus Creator/2  "I0"
  Convert2/1 -> Bus Creator/3  "Q1"
  Convert3/1 -> Bus Creator/4  "I1"
  Gateway Out6/1 -> DAC drive/1
  Gateway Out7/1 -> DAC drive/2
  Gateway Out8/1 -> DAC drive/3
  Gateway Out9/1 -> DAC drive/4
  Mux/1 -> Scope/1
  Gateway Out/1 -> Mux/1
  Gateway Out2/1 -> Mux/2
  Gateway Out1/1 -> Mux1/1
  Gateway Out3/1 -> Mux1/2
  Mux1/1 -> Scope/2
  Shift/1 -> DDS Compiler 6.0 1/2

== system CryoDetXray/DspCore/DAC format/DAC demux clock ==
  note: Use DAC clock to generate edge to synchronize simulation of DAC demuxing in FPGA VHDL wrapper
      | output 1 = I
      | 0 = Q
      | This generates no code in FPGA, it is just  here to make Simulink simulation run
  In1 : Inport
  Add : Sum
  Clock Enable Probe : xbsIndex_r4/Clock Enable Probe  inherit_constraints=on  block_type=ceprobe
      settings: infoedit="Clock enable extractor.  Produces a Boolean output that mirrors the hardware clock enable associated with the input sample rate.<br><br>Hardware notes: in hardware this block costs nothing."
  Constant : Constant  Value=2
  Down Sample : xbsIndex_r4/Down Sample  sample_ratio=2  sample_phase="Last Value of Frame  (most efficient)"  en=off  rst=off  latency=1  dbl_ovrd=off  block_type=dsamp
  Interleaver Scope : Scope  NumInputPorts=3
  Math Function : Math  Operator=mod  SaturateOnIntegerOverflow=on
  Transport Delay : TransportDelay  DelayTime=Tclk/2
  fromdsp_dacdata1_2 : xbsIndex_r4/Gateway Out  inherit_from_input=off  hdl_port=off  rows=1  columns=1  UseAsDAC=off  DACChannel='1'  interface=None  automatic_assignment=on  address_offset=hex2dec('00')  intf_name=''  intf_description=''  timing_constraint=None  locs_specified=off  LOCs={}  io_standard={}  block_type=gatewayout
  IQtoggle : Outport
  wires:
  Clock Enable Probe/1 -> fromdsp_dacdata1_2/1
  Down Sample/1 -> Clock Enable Probe/1
  In1/1 -> Down Sample/1
  fromdsp_dacdata1_2/1 -> Interleaver Scope/1, Add/1, Transport Delay/1
  Transport Delay/1 -> Add/2
  Math Function/1 -> Interleaver Scope/3, IQtoggle/1
  Constant/1 -> Math Function/2
  Add/1 -> Interleaver Scope/2, Math Function/1

== system CryoDetXray/DspCore/AdcDac 0/16LineUDC 0/DAC Sum ==
  note: Sum I0, Q0, I1, Q1 across all 16 input channels
  note: Changed from 12 channel to 16 channels 8Sept2017
  In1 : Inport
  In2 : Inport  Port=2
  In3 : Inport  Port=3
  In4 : Inport  Port=4
  In5 : Inport  Port=5
  In6 : Inport  Port=6
  In7 : Inport  Port=7
  In8 : Inport  Port=8
  In9 : Inport  Port=9
  In10 : Inport  Port=10
  In11 : Inport  Port=11
  In12 : Inport  Port=12
  In13 : Inport  Port=13
  In14 : Inport  Port=14
  In15 : Inport  Port=15
  In16 : Inport  Port=16
  Bus Creator : BusCreator  Inputs=4
  Bus Creator1 : BusCreator  Inputs=16
  DAC Q0 SUM : Subsystem
  DAC Q1 SUM : Subsystem
  DAC i0 SUM : Subsystem
  DAC i1 SUM : Subsystem
  Gateway Out{,1..3} (4 alike) : xbsIndex_r4/Gateway Out  Commented=on  inherit_from_input=off  hdl_port=off  rows=1  columns=1  UseAsDAC=off  DACChannel='1'  interface=None  automatic_assignment=on  address_offset=hex2dec('00')  intf_name=''  intf_description=''  timing_constraint=None  locs_specified=off  LOCs={}  io_standard={}  block_type=gatewayout
  Scope : Scope  Commented=on  NumInputPorts=4
  Out1 : Outport
  wires:
  In3/1 -> Bus Creator1/3
  In4/1 -> Bus Creator1/4
  In5/1 -> Bus Creator1/5
  In6/1 -> Bus Creator1/6
  In7/1 -> Bus Creator1/7
  In8/1 -> Bus Creator1/8
  In9/1 -> Bus Creator1/9
  In11/1 -> Bus Creator1/11
  In12/1 -> Bus Creator1/12
  In13/1 -> Bus Creator1/13
  In14/1 -> Bus Creator1/14
  In15/1 -> Bus Creator1/15
  In16/1 -> Bus Creator1/16
  In2/1 -> Bus Creator1/2
  In1/1 -> Bus Creator1/1
  In10/1 -> Bus Creator1/10
  Bus Creator1/1 -> DAC i1 SUM/1(In1), DAC Q1 SUM/1(In1), DAC Q0 SUM/1(In1), DAC i0 SUM/1(In1)
  DAC Q0 SUM/1(Out1) -> Gateway Out/1, Bus Creator/1  "Q0 sum"
  DAC i0 SUM/1(Out1) -> Gateway Out1/1, Bus Creator/2  "I0 sum"
  DAC Q1 SUM/1(Out1) -> Gateway Out2/1, Bus Creator/3  "Q1 sum"
  DAC i1 SUM/1(Out1) -> Gateway Out3/1, Bus Creator/4  "I1 sum"
  Bus Creator/1 -> Out1/1
  Gateway Out/1 -> Scope/1
  Gateway Out1/1 -> Scope/2
  Gateway Out2/1 -> Scope/3
  Gateway Out3/1 -> Scope/4

== system CryoDetXray/DspCore/AdcDac 0/16LineUDC 0/Mux16X4 ==
  note: I think this will select a channel 1 or 2 ticks after it has updated,
      | which should work fine. But optimal would be to delay synch in by 11 ticks = N-1
  note: Channel ID
  note: Reference Q&I
  note: Signal Q&I
  note: Sixteen busses 4-wide each time-division multiplexed onto a 4-wide bus
  synch : Inport
  line0 : Inport  Port=2
  line1 : Inport  Port=3
  line2 : Inport  Port=4
  line3 : Inport  Port=5
  line4 : Inport  Port=6
  line5 : Inport  Port=7
  line6 : Inport  Port=8
  line7 : Inport  Port=9
  line8 : Inport  Port=10
  line9 : Inport  Port=11
  line10 : Inport  Port=12
  line11 : Inport  Port=13
  line12 : Inport  Port=14
  line13 : Inport  Port=15
  line14 : Inport  Port=16
  line15 : Inport  Port=17
  Bus Creator{,1..3} (4 alike) : BusCreator  Inputs=2
  Counter : xbsIndex_r4/Counter  cnt_type=Count Limited  cnt_to=15  operation=Up  start_count=0  cnt_by_val=1  arith_type=Unsigned  n_bits=4  bin_pt=0  load_pin=off  rst=on  en=off  explicit_period=off  period=Tclk  use_behavioral_HDL=off  implementation=Fabric  dbl_ovrd=off  block_type=counter
  Delay1 : xbsIndex_r4/Delay  rst=off  infoeditControl=Selection of Reset will increase slice count due to use of real FFs and instead of SRLs  en=off  latency=1  reg_retiming=off  dbl_ovrd=off  block_type=delay
  Demux{,1..15} (16 alike) : Demux
  Mux{,1..3} (4 alike) : xbsIndex_r4/Mux  inputs=16  en=off  latency=1  precision=Full  arith_type=Unsigned  n_bits=16  bin_pt=14  quantization=Truncate  overflow=Wrap  dbl_ovrd=off  block_type=mux
  Out1 : Outport
  wires:
  line0/1 -> Demux/1
  line5/1 -> Demux6/1
  line4/1 -> Demux5/1
  line3/1 -> Demux4/1
  line2/1 -> Demux3/1
  line1/1 -> Demux1/1
  Demux/1 -> Mux/2
  Demux/2 -> Mux1/2
  Demux/3 -> Mux2/2
  Demux/4 -> Mux3/2
  Demux1/1 -> Mux/3
  Demux1/2 -> Mux1/3
  Demux1/3 -> Mux2/3
  Demux1/4 -> Mux3/3
  Demux3/1 -> Mux/4
  Demux3/2 -> Mux1/4
  Demux3/3 -> Mux2/4
  Demux3/4 -> Mux3/4
  Demux4/1 -> Mux/5
  Demux4/2 -> Mux1/5
  Demux4/3 -> Mux2/5
  Demux4/4 -> Mux3/5
  Demux5/1 -> Mux/6
  Demux5/2 -> Mux1/6
  Demux5/3 -> Mux2/6
  Demux5/4 -> Mux3/6
  Demux6/1 -> Mux/7
  Demux6/2 -> Mux1/7
  Demux6/3 -> Mux2/7
  Demux6/4 -> Mux3/7
  synch/1 -> Counter/1
  Mux/1 -> Bus Creator1/1  "sigQ"
  Mux1/1 -> Bus Creator1/2  "sigI"
  Mux2/1 -> Bus Creator2/1  "refQ"
  Mux3/1 -> Bus Creator2/2  "refI"
  Bus Creator1/1 -> Bus Creator3/1  "SignalQ&I"
  Bus Creator2/1 -> Bus Creator3/2  "ReferenceQ&I"
  Counter/1 -> Mux2/1, Delay1/1, Mux1/1, Mux3/1, Mux/1
  Bus Creator3/1 -> Bus Creator/2  "Sig&Ref"
  Delay1/1 -> Bus Creator/1  "channel"
  Bus Creator/1 -> Out1/1
  line8/1 -> Demux2/1
  line9/1 -> Demux7/1
  line10/1 -> Demux8/1
  line11/1 -> Demux9/1
  line12/1 -> Demux10/1
  line13/1 -> Demux11/1
  line7/1 -> Demux13/1
  line6/1 -> Demux12/1
  line14/1 -> Demux14/1
  line15/1 -> Demux15/1
  Demux14/3 -> Mux2/16
  Demux12/1 -> Mux/8
  Demux12/2 -> Mux1/8
  Demux12/3 -> Mux2/8
  Demux12/4 -> Mux3/8
  Demux13/1 -> Mux/9
  Demux13/2 -> Mux1/9
  Demux13/3 -> Mux2/9
  Demux13/4 -> Mux3/9
  Demux2/1 -> Mux/10
  Demux2/2 -> Mux1/10
  Demux2/3 -> Mux2/10
  Demux2/4 -> Mux3/10
  Demux7/1 -> Mux/11
  Demux7/2 -> Mux1/11
  Demux7/3 -> Mux2/11
  Demux7/4 -> Mux3/11
  Demux8/1 -> Mux/12
  Demux8/2 -> Mux1/12
  Demux8/3 -> Mux2/12
  Demux8/4 -> Mux3/12
  Demux9/1 -> Mux/13
  Demux9/2 -> Mux1/13
  Demux9/3 -> Mux2/13
  Demux9/4 -> Mux3/13
  Demux10/1 -> Mux/14
  Demux10/2 -> Mux1/14
  Demux10/3 -> Mux2/14
  Demux10/4 -> Mux3/14
  Demux11/1 -> Mux/15
  Demux11/2 -> Mux1/15
  Demux11/3 -> Mux2/15
  Demux11/4 -> Mux3/15
  Demux14/1 -> Mux/16
  Demux14/2 -> Mux1/16
  Demux14/4 -> Mux3/16
  Demux15/1 -> Mux/17
  Demux15/2 -> Mux1/17
  Demux15/3 -> Mux2/17
  Demux15/4 -> Mux3/17
